simulink model "ASW"  (R2014a)
settings: Solver=FixedStepDiscrete  StartTime=0.0  StopTime=10.0  FixedStep=0.0001  RelTol=1e-3
settings Model: Creator=HP  LastModifiedBy=HP
settings OptimizationCC: InlineParams=on  OptimizeModelRefInitCode=on  LifeSpan=1
settings RTWCC: SystemTargetFile=ert.tlc  TemplateMakefile=ert_default_tmf  Description=Embedded Coder  GenerateReport=on  ProcessScript=ert_make_rtw_hook  IncludeHyperlinkInReport=on  LaunchReport=on
settings CodeAppCC: IgnoreCustomStorageClasses=off
settings ERTTargetCC: ParMdlRefBuildCompliant=on  CompOptLevelCompliant=on  ConcurrentExecutionCompliant=on  ERTFirstTimeCompliant=on  ModelStepFunctionPrototypeControlCompliant=on  CPPClassGenCompliant=on  InlinedParameterPlacement=Hierarchical  ERTCustomFileTemplate=example_file_process.tlc

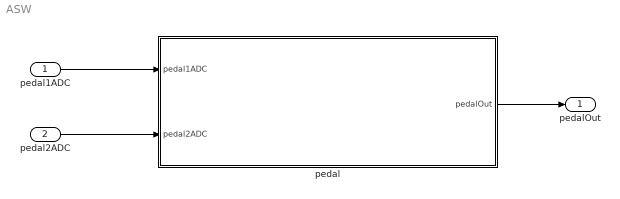
== system ASW ==
  pedal1ADC : Inport
  pedal2ADC : Inport  Port=2
  pedal : Subsystem  TreatAsAtomicUnit=on  RTWFcnName=pedal  RTWFileName=pedal
      settings: RTWSystemCode=Nonreusable function  RTWFcnNameOpts=User specified  RTWFileNameOpts=User specified  FunctionInterfaceSpec=Allow arguments  FunctionWithSeparateData=on
  pedalOut : Outport
  wires:
  pedal1ADC/1 -> pedal/1(pedal1ADC)
  pedal2ADC/1 -> pedal/2(pedal2ADC)
  pedal/1(pedalOut) -> pedalOut/1

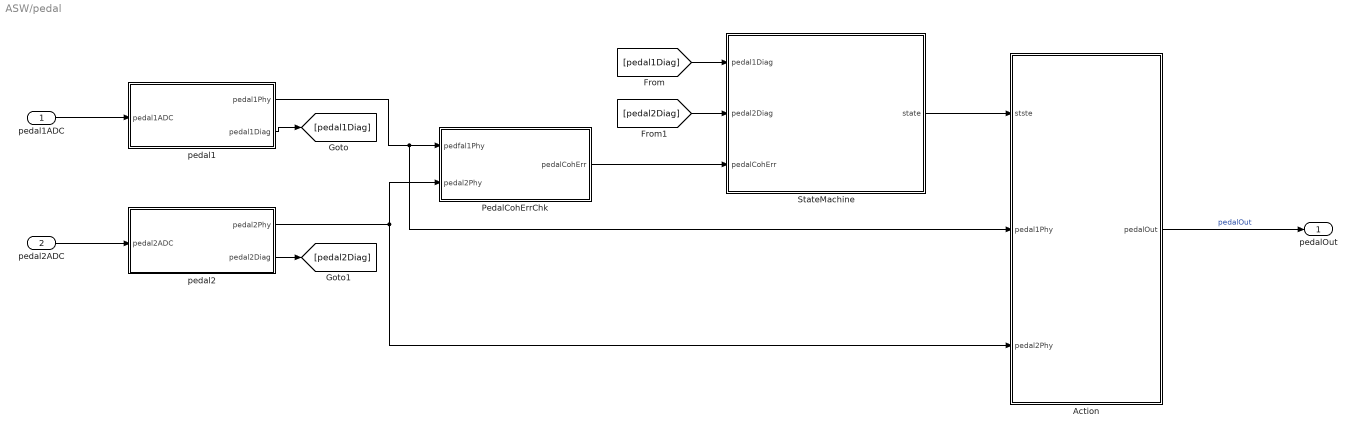
== system ASW/pedal ==
  pedal1ADC : Inport
  pedal2ADC : Inport  Port=2
  Action : Subsystem
  PedalCohErrChk : Subsystem
  StateMachine : Subsystem
  pedal1 : Subsystem
  pedal2 : Subsystem
  pedalOut : Outport
  wires:
  [pedal1Diag] -> StateMachine/1(pedal1Diag)
  PedalCohErrChk/1(pedalCohErr) -> StateMachine/3(pedalCohErr)
  pedal2/2(pedal2Diag) -> [pedal2Diag]
  pedal1/2(pedal1Diag) -> [pedal1Diag]
  [pedal2Diag] -> StateMachine/2(pedal2Diag)
  pedal1/1(pedal1Phy) -> Action/2(pedal1Phy), PedalCohErrChk/1(pedfal1Phy)
  pedal2/1(pedal2Phy) -> Action/3(pedal2Phy), PedalCohErrChk/2(pedal2Phy)
  pedal1ADC/1 -> pedal1/1(pedal1ADC)
  pedal2ADC/1 -> pedal2/1(pedal2ADC)
  Action/1(pedalOut) -> pedalOut/1  "pedalOut"
  StateMachine/1(state) -> Action/1(stste)

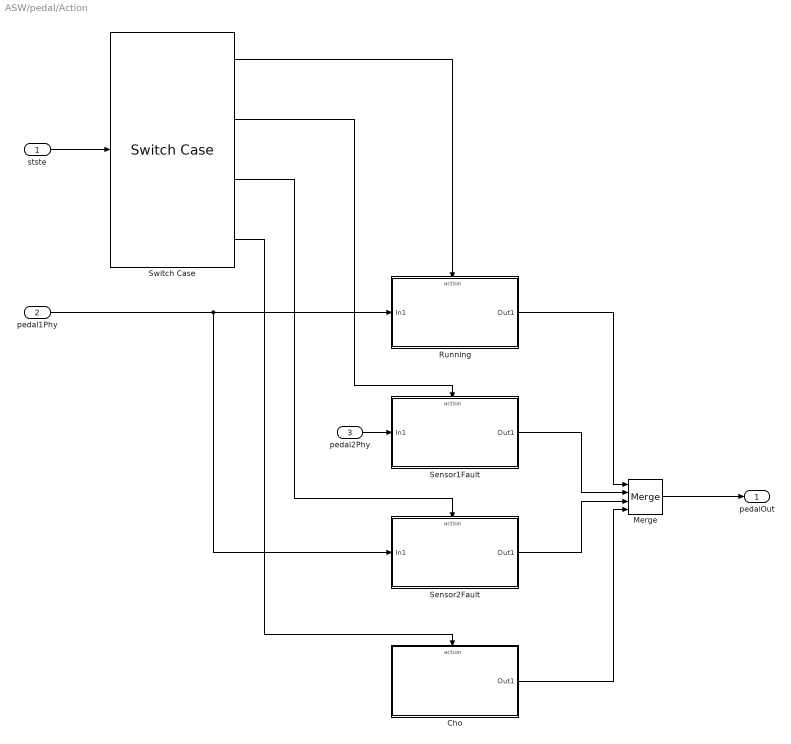
== system ASW/pedal/Action ==
  stste : Inport
  pedal1Phy : Inport  Port=2
  pedal2Phy : Inport  Port=3
  Cho : Subsystem  TreatAsAtomicUnit=on
  Merge : Merge  Inputs=4
  Running : Subsystem  TreatAsAtomicUnit=on
  Sensor1Fault : Subsystem  TreatAsAtomicUnit=on
  Sensor2Fault : Subsystem  TreatAsAtomicUnit=on
  Switch Case : SwitchCase  CaseConditions={0, 1, 2, 3}  ShowDefaultCase=off
  pedalOut : Outport
  wires:
  Switch Case/1 -> Running/Action
  Switch Case/2 -> Sensor1Fault/Action
  Switch Case/4 -> Cho/Action
  Switch Case/3 -> Sensor2Fault/Action
  stste/1 -> Switch Case/1
  Running/1(Out1) -> Merge/1
  Cho/1(Out1) -> Merge/4
  Sensor1Fault/1(Out1) -> Merge/2
  Sensor2Fault/1(Out1) -> Merge/3
  pedal2Phy/1 -> Sensor1Fault/1(In1)
  pedal1Phy/1 -> Sensor2Fault/1(In1), Running/1(In1)
  Merge/1 -> pedalOut/1

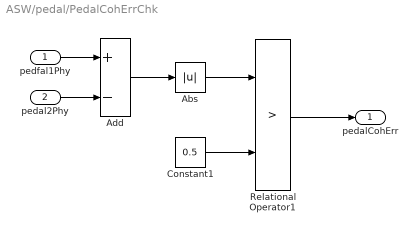
== system ASW/pedal/PedalCohErrChk ==
  pedfal1Phy : Inport
  pedal2Phy : Inport  Port=2
  Abs : Abs
  Add : Sum  Inputs=+-
  Constant1 : Constant  Value=0.5  OutDataTypeStr=single
  Relational Operator1 : RelationalOperator  Operator=>  OutDataTypeStr=boolean
  pedalCohErr : Outport
  wires:
  Relational Operator1/1 -> pedalCohErr/1
  pedfal1Phy/1 -> Add/1
  Add/1 -> Abs/1
  pedal2Phy/1 -> Add/2
  Constant1/1 -> Relational Operator1/2
  Abs/1 -> Relational Operator1/1

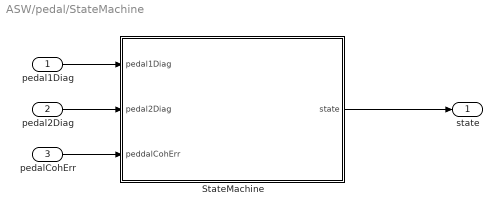
== system ASW/pedal/StateMachine ==
  pedal1Diag : Inport
  pedal2Diag : Inport  Port=2
  pedalCohErr : Inport  Port=3
  StateMachine : Stateflow chart  TreatAsAtomicUnit=on
  state : Outport
  wires:
  pedalCohErr/1 -> StateMachine/3(peddalCohErr)
  StateMachine/1(state) -> state/1
  pedal2Diag/1 -> StateMachine/2(pedal2Diag)
  pedal1Diag/1 -> StateMachine/1(pedal1Diag)

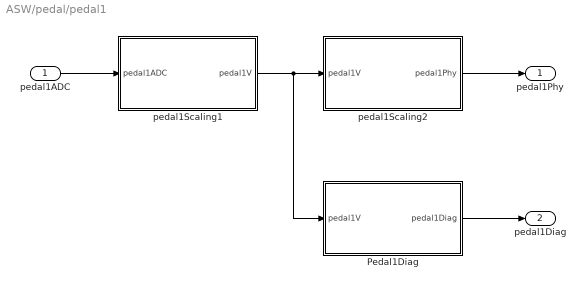
== system ASW/pedal/pedal1 ==
  pedal1ADC : Inport
  Pedal1Diag : Subsystem
  pedal1Scaling1 : Subsystem
  pedal1Scaling2 : Subsystem
  pedal1Phy : Outport
  pedal1Diag : Outport  Port=2
  wires:
  pedal1Scaling1/1(pedal1V) -> pedal1Scaling2/1(pedal1V), Pedal1Diag/1(pedal1V)
  pedal1Scaling2/1(pedal1Phy) -> pedal1Phy/1
  Pedal1Diag/1(pedal1Diag) -> pedal1Diag/1
  pedal1ADC/1 -> pedal1Scaling1/1(pedal1ADC)

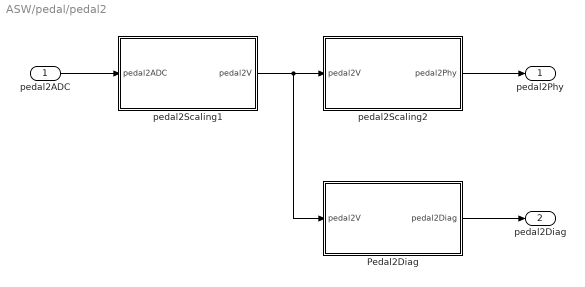
== system ASW/pedal/pedal2 ==
  pedal2ADC : Inport
  Pedal2Diag : Subsystem
  pedal2Scaling1 : Subsystem
  pedal2Scaling2 : Subsystem
  pedal2Phy : Outport
  pedal2Diag : Outport  Port=2
  wires:
  pedal2ADC/1 -> pedal2Scaling1/1(pedal2ADC)
  Pedal2Diag/1(pedal2Diag) -> pedal2Diag/1
  pedal2Scaling2/1(pedal2Phy) -> pedal2Phy/1
  pedal2Scaling1/1(pedal2V) -> Pedal2Diag/1(pedal2V), pedal2Scaling2/1(pedal2V)

== system ASW/pedal/Action/Cho ==
  Action Port : ActionPort  ActionType=case
  Constant1 : Constant  Value=0  OutDataTypeStr=single
  Out1 : Outport
  wires:
  Constant1/1 -> Out1/1

== system ASW/pedal/Action/Running ==
  In1 : Inport
  Action Port : ActionPort  ActionType=case
  Out1 : Outport
  wires:
  In1/1 -> Out1/1

== system ASW/pedal/Action/Sensor1Fault ==
  In1 : Inport
  Action Port : ActionPort  ActionType=case
  Saturation : Saturate  UpperLimit=20  LowerLimit=0
  Out1 : Outport
  wires:
  In1/1 -> Saturation/1
  Saturation/1 -> Out1/1

== system ASW/pedal/Action/Sensor2Fault ==
  In1 : Inport
  Action Port : ActionPort  ActionType=case
  Saturation : Saturate  UpperLimit=20  LowerLimit=0
  Out1 : Outport
  wires:
  Saturation/1 -> Out1/1
  In1/1 -> Saturation/1

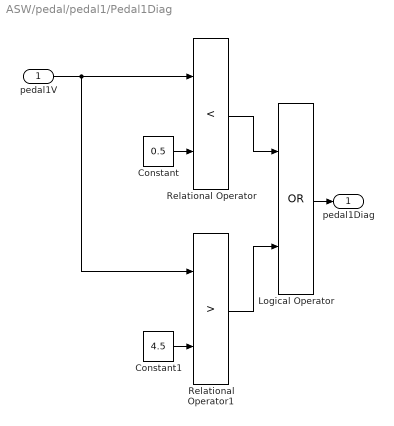
== system ASW/pedal/pedal1/Pedal1Diag ==
  pedal1V : Inport
  Constant : Constant  Value=0.5  OutDataTypeStr=single
  Constant1 : Constant  Value=4.5  OutDataTypeStr=single
  Logical Operator : Logic  Operator=OR  AllPortsSameDT=off  OutDataTypeStr=boolean
  Relational Operator : RelationalOperator  Operator=<  OutDataTypeStr=boolean
  Relational Operator1 : RelationalOperator  Operator=>  OutDataTypeStr=boolean
  pedal1Diag : Outport
  wires:
  Logical Operator/1 -> pedal1Diag/1
  Relational Operator/1 -> Logical Operator/1
  Constant1/1 -> Relational Operator1/2
  pedal1V/1 -> Relational Operator1/1, Relational Operator/1
  Relational Operator1/1 -> Logical Operator/2
  Constant/1 -> Relational Operator/2

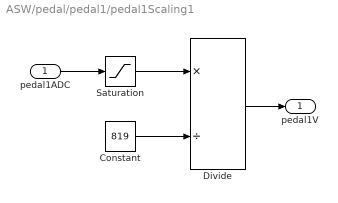
== system ASW/pedal/pedal1/pedal1Scaling1 ==
  pedal1ADC : Inport
  Constant : Constant  Value=819  OutDataTypeStr=uint16
  Divide : Product  Inputs=*/  OutDataTypeStr=single
  Saturation : Saturate  UpperLimit=4095  LowerLimit=0  OutDataTypeStr=uint16
  pedal1V : Outport
  wires:
  Constant/1 -> Divide/2
  Divide/1 -> pedal1V/1
  pedal1ADC/1 -> Saturation/1
  Saturation/1 -> Divide/1

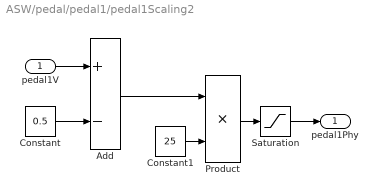
== system ASW/pedal/pedal1/pedal1Scaling2 ==
  pedal1V : Inport
  Add : Sum  Inputs=+-
  Constant : Constant  Value=0.5  OutDataTypeStr=single
  Constant1 : Constant  Value=25  OutDataTypeStr=single
  Product : Product
  Saturation : Saturate  UpperLimit=100  LowerLimit=0  OutDataTypeStr=single
  pedal1Phy : Outport
  wires:
  Constant/1 -> Add/2
  pedal1V/1 -> Add/1
  Constant1/1 -> Product/2
  Product/1 -> Saturation/1
  Add/1 -> Product/1
  Saturation/1 -> pedal1Phy/1

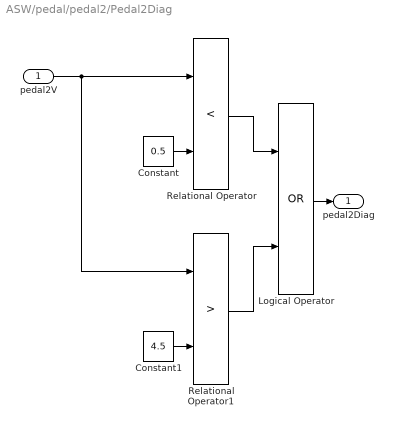
== system ASW/pedal/pedal2/Pedal2Diag ==
  pedal2V : Inport
  Constant : Constant  Value=0.5  OutDataTypeStr=single
  Constant1 : Constant  Value=4.5  OutDataTypeStr=single
  Logical Operator : Logic  Operator=OR  AllPortsSameDT=off  OutDataTypeStr=boolean
  Relational Operator : RelationalOperator  Operator=<  OutDataTypeStr=boolean
  Relational Operator1 : RelationalOperator  Operator=>  OutDataTypeStr=boolean
  pedal2Diag : Outport
  wires:
  Constant/1 -> Relational Operator/2
  Relational Operator1/1 -> Logical Operator/2
  pedal2V/1 -> Relational Operator/1, Relational Operator1/1
  Constant1/1 -> Relational Operator1/2
  Relational Operator/1 -> Logical Operator/1
  Logical Operator/1 -> pedal2Diag/1

== system ASW/pedal/pedal2/pedal2Scaling1 ==
  pedal2ADC : Inport
  Constant : Constant  Value=819  OutDataTypeStr=uint16
  Divide : Product  Inputs=*/  OutDataTypeStr=single
  Saturation : Saturate  UpperLimit=4095  LowerLimit=0  OutDataTypeStr=uint16
  pedal2V : Outport
  wires:
  Saturation/1 -> Divide/1
  pedal2ADC/1 -> Saturation/1
  Divide/1 -> pedal2V/1
  Constant/1 -> Divide/2

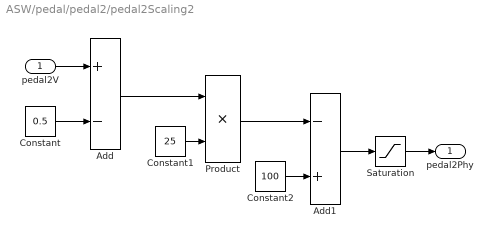
== system ASW/pedal/pedal2/pedal2Scaling2 ==
  pedal2V : Inport
  Add : Sum  Inputs=+-
  Add1 : Sum  Inputs=-+
  Constant : Constant  Value=0.5  OutDataTypeStr=single
  Constant1 : Constant  Value=25  OutDataTypeStr=single
  Constant2 : Constant  Value=100  OutDataTypeStr=single
  Product : Product
  Saturation : Saturate  UpperLimit=100  LowerLimit=0  OutDataTypeStr=single
  pedal2Phy : Outport
  wires:
  Saturation/1 -> pedal2Phy/1
  Add/1 -> Product/1
  Constant1/1 -> Product/2
  pedal2V/1 -> Add/1
  Constant/1 -> Add/2
  Product/1 -> Add1/1
  Constant2/1 -> Add1/2
  Add1/1 -> Saturation/1

== stateflow chart ASW/pedal/StateMachine/StateMachine ==
  state Running
    entry: state = uint8(0);
  state Sensor2Fault
    entry: state = uint8(2);
  state Sensor1Fault
    entry: state = uint8(1);
  state COH
    entry: state = uint8(3);
  (default) -> Running
  (junction 6) -> Running [order 5]
  Running -> (junction 6)
  (junction 6) -> Sensor2Fault [order 3] : [pedal2Diag]
  (junction 6) -> Sensor1Fault [order 2] : [pedal1Diag]
  Sensor2Fault -> (junction 6)
  Sensor1Fault -> (junction 6)
  (junction 6) -> COH [order 4] : [peddalCohErr]
  (junction 6) -> COH [order 1] : [pedal1Diag&&pedal2Diag]
  COH -> (junction 6)
  data: pedal1Diag input boolean size=1 [0..1]; pedal2Diag input boolean size=1 [0..1]; peddalCohErr input boolean size=1 [0..1]; state output uint8 size=1 [0..5]
